simulink model "imgBB"  (R2020a)
settings: Solver=FixedStepAuto  StartTime=0.0  StopTime=10.0  RelTol=1e-3
undefined symbols (not defined in the file): blue, green, red
libraries: androiduilib x1, androidaudiovideolib x1
settings Model: Creator=luisi  LastModifiedBy=luisi
settings OptimizationCC: EnhancedBackFolding=on  PassReuseOutputArgsAs=Individual arguments  ZeroExternalMemoryAtStartup=off  ZeroInternalMemoryAtStartup=off  MaxStackSize=64  OptimizeBlockOrder=speed  DifferentSizesBufferReuse=on  OptimizationCustomize=off  EfficientTunableParamExpr=on
settings DebuggingCC: ParameterTunabilityLossMsg=error
settings HardwareCC: ProdBitPerPointer=32  ProdBitPerSizeT=32  ProdBitPerPtrDiffT=32  ProdLargestAtomicInteger=Long  ProdLargestAtomicFloat=Double  ProdWordSize=32  ProdHWDeviceType=ARM Compatible->ARM Cortex
settings SFSimCC: MATLABDynamicMemAlloc=off
settings RTWCC: SystemTargetFile=ert.tlc  HardwareBoard=Android Device  TemplateMakefile=ert_default_tmf  RTWVerbose=off  Toolchain=Android SDK/NDK Tools
settings CodeAppCC: ForceParamTrailComments=on  IgnoreCustomStorageClasses=off  OperatorAnnotations=on  SimulinkDataObjDesc=on  SFDataObjDesc=on  InsertBlockDesc=on
settings ERTTargetCC: ExtModeMexArgs='192.168.0.149'

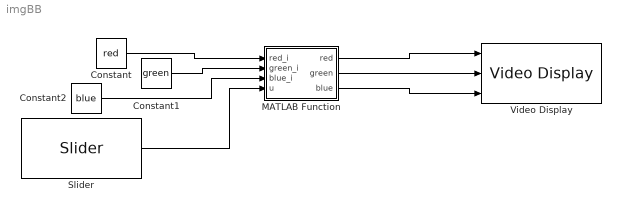
== system imgBB ==
  Constant : Constant  Value=red
  Constant1 : Constant  Value=green
  Constant2 : Constant  Value=blue
  MATLAB Function : MATLAB Function  TreatAsAtomicUnit=on
  Slider : androiduilib/Slider  Min=0  Value=0  Max=2  Resolution=1  SliderId=imgBB/Slider  SampleTime=0.1  BlockPlatform=Android
      settings: SourceProductBaseCode=ANDROID
  Video Display : androidaudiovideolib/Video Display  BlockPlatform=Android
      settings: SourceProductBaseCode=ANDROID
  wires:
  MATLAB Function/3(blue) -> Video Display/3
  Constant2/1 -> MATLAB Function/3(blue_i)
  Slider/1 -> MATLAB Function/4(u)
  Constant1/1 -> MATLAB Function/2(green_i)
  Constant/1 -> MATLAB Function/1(red_i)
  MATLAB Function/2(green) -> Video Display/2
  MATLAB Function/1(red) -> Video Display/1

== matlab function imgBB/MATLAB Function ==
  data: red_i input; green_i input; red output; green output; blue_i input; u input; blue output
function [red, green, blue] = fcn(red_i, green_i,blue_i,u)
    frio =205;
    fiebre=600;
    if u==0 %normal
        blue=blue_i;
        red=red_i;
        green=green_i;
        
    elseif u==1 %fiebre
        
        %cachete izq
        for c= 430:550
            for m=550:700
                red_i(c,m)= fiebre;
            end
        end
        %cachete derecho
        for c= 470:600
            for m=300:400
                red_i(c,m)=fiebre;
                
            end
        end
        %labios
        for c= 550:600
            for m=440:530
                red_i(c,m)=fiebre;
            end
        end
        blue=blue_i;
        red=red_i;
        green=green_i;
    else
        %frio
          %cachete izq
        for c= 430:550
            for m=550:700
                blue_i(c,m)=frio;
                
            end
        end
        %cachete derecho
        for c= 470:600
            for m=300:400
                blue_i(c,m)=frio;
                %redcalor(c,m)=calor;
            end
        end
        %labios
        for c= 550:600
            for m=440:530
                blue_i(c,m)=frio;
                %redcalor(c,m)=380;
            end
        end
        blue=blue_i;
        red=red_i;
        green=green_i;
    end
